simulink model "PID_SERVO_SG90"  (R2023a)
settings: Solver=FixedStepAuto  StartTime=0.0  StopTime=inf  FixedStep=0.001  RelTol=1e-3
libraries: arduinolib x2, simulink x1
settings Model: ExtModeTrigDuration=2  Creator=Mario  LastModifiedBy=Mario
settings OptimizationCC: EnhancedBackFolding=on  PassReuseOutputArgsAs=Individual arguments  ZeroExternalMemoryAtStartup=off  ZeroInternalMemoryAtStartup=off  MaxStackSize=64  OptimizeBlockOrder=speed  DifferentSizesBufferReuse=on  OptimizationCustomize=off  EfficientTunableParamExpr=on
settings DebuggingCC: ParameterPrecisionLossMsg=none  ParameterTunabilityLossMsg=error
settings HardwareCC: ProdBitPerPointer=32  ProdBitPerSizeT=32  ProdBitPerPtrDiffT=32  ProdLargestAtomicInteger=Long  ProdLargestAtomicFloat=Double  ProdWordSize=32  ProdHWDeviceType=ARM Compatible->ARM Cortex  UseEmbeddedCoderFeatures=off
settings SFSimCC: MATLABDynamicMemAlloc=off
settings RTWCC: Description=Embedded Coder  SystemTargetFile=ert.tlc  HardwareBoard=Arduino Due  TemplateMakefile=ert_default_tmf  Toolchain=Arduino ARM  BuildConfiguration=Faster Runs
settings CodeAppCC: ForceParamTrailComments=on  IgnoreCustomStorageClasses=off  OperatorAnnotations=on  SimulinkDataObjDesc=on  SFDataObjDesc=on  InsertBlockDesc=on
settings ERTTargetCC: SupportContinuousTime=on  SupportNonInlinedSFcns=on  SupportVariableSizeSignals=on  ExtModeTransport=3  ExtModeStaticAlloc=on  ExtModeAutomaticAllocSize=off  ExtModeStaticAllocSize=24576  ExtModeMexFile=ext_xcp  ExtModeIntrfLevel=Level2 - Open

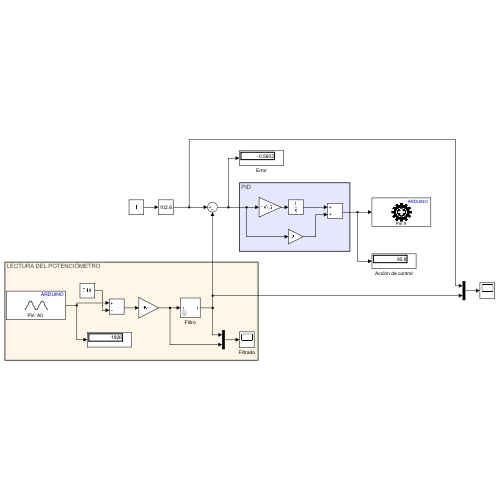
[thumbnail: Simulink's stored preview of the top-level diagram]
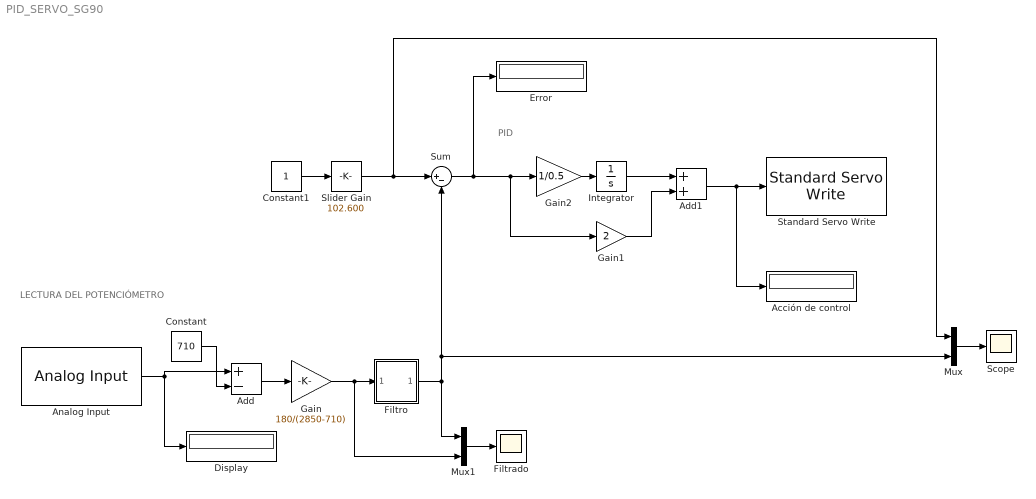
== system PID_SERVO_SG90 ==
  note: LECTURA DEL POTENCIÓMETRO
  note: PID
  Acción de control : Display
  Add : Sum  Inputs=+-
  Add1 : Sum
  Analog Input : arduinolib/Analog Input  pinNumber=0  ReadResultsOnly=off  ConversionTriggerSource=Software  ExternalTriggerType=uint32( 0 )  OutputDataType=uint16  EnableConversionCompleteNotify=off  EnableOuputStatus=off  SampleTime=-1  blockPlatform=arduino
  Constant : Constant  Value=710
  Constant1 : Constant
  Display : Display
  Error : Display
  Filtrado : Scope
  Filtro : Subsystem  mask{AlfaPar=0.01}
      mask prompts: AlfaPar "alfa"
  Gain : Gain  Gain=180/(2850-710)
  Gain1 : Gain  Gain=2
  Gain2 : Gain  Gain=1/0.5
  Integrator : Integrator
  Mux : Mux  Inputs=2
  Mux1 : Mux  Inputs=2
  Scope : Scope
  Slider Gain : simulink/Math Operations/Slider Gain  gain=102.600  low=0  high=180
  Standard Servo Write : arduinolib/Standard Servo Write  pinNumber=9  ServoIndex=0  blockPlatform=ARDUINO
  Sum : Sum  Inputs=|+-
  wires:
  Analog Input/1 -> Add/1, Display/1
  Constant/1 -> Add/2
  Add/1 -> Gain/1
  Gain2/1 -> Integrator/1
  Integrator/1 -> Add1/1
  Gain1/1 -> Add1/2
  Add1/1 -> Acción de control/1, Standard Servo Write/1
  Constant1/1 -> Slider Gain/1
  Slider Gain/1 -> Mux/1, Sum/1
  Sum/1 -> Error/1, Gain2/1, Gain1/1
  Mux/1 -> Scope/1
  Filtro/1(Output) -> Mux1/1, Mux/2, Sum/2
  Mux1/1 -> Filtrado/1
  Gain/1 -> Mux1/2, Filtro/1(In1)

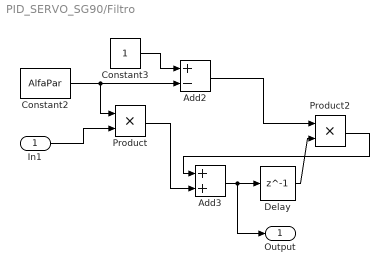
== system PID_SERVO_SG90/Filtro ==
  In1 : Inport
  Add2 : Sum  Inputs=+-
  Add3 : Sum
  Constant2 : Constant  Value=AlfaPar
  Constant3 : Constant
  Delay : Delay  DelayLength=1
  Product : Product
  Product2 : Product
  Output : Outport
  wires:
  In1/1 -> Product/2
  Add3/1 -> Output/1, Delay/1
  Delay/1 -> Product2/2
  Product2/1 -> Add3/1
  Constant3/1 -> Add2/1
  Constant2/1 -> Add2/2, Product/1
  Add2/1 -> Product2/1
  Product/1 -> Add3/2
